simulink library "T_Sensor_Surface"  (Simulink 8.2)
settings: Solver=ode45  StartTime=0.0  StopTime=10.0  RelTol=1e-3
settings Model: Creator=lena.frank  LastModifiedBy=drhf

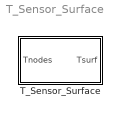
== system T_Sensor_Surface ==
  T_Sensor_Surface : Subsystem  mask(surface temperature sensor){pos=[0.1 0.4 0.5 0.9], tdel=1, t0=20}
      mask prompts: pos "relative position 0..1 (0 = bottom, 1 = top)"; tdel "delay-time in s"; t0 "initial temperature in degree centigrade"
      mask help:
      | Surface temperature sensor for a storage. The block breaks the algebraic loop when connecting the node temperature directly to the controller.
      | The relative position can be a vector for several sensors, for example [0.1 0.5 0.9]
      mask init:
      | tdel = max(tdel,0.01);
      | pos = max(0, min(pos, 1));
      mask Help: web(fullfile(path_carnot('help'),'T_Sensor_Surface.html'),'-helpbrowser')
      mask Display: plot(-10,0,110,100,[50,55,65,70,70,65,55,45,35,30,30,35,44,50,50],[50,50,60,70,80,90,100,100,90,80,70,60,50,50,-0],[60,40],[90,90],[50,50],[57,90])

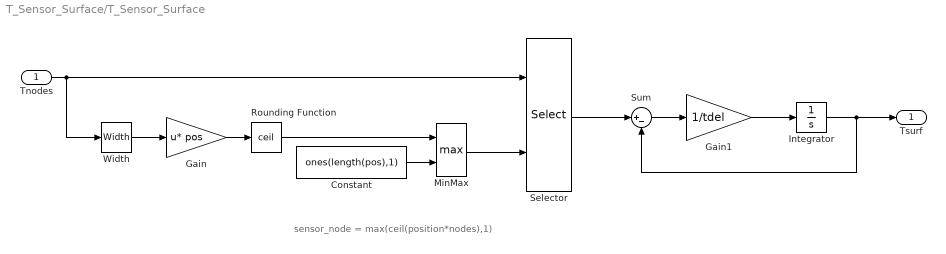
== system T_Sensor_Surface/T_Sensor_Surface ==
  note: sensor_node = max(ceil(position*nodes),1)
  Tnodes : Inport
  Constant : Constant  Value=ones(length(pos),1)
  Gain : Gain  Gain=pos  Multiplication=Matrix(u*K)
  Gain1 : Gain  Gain=1/tdel
  Integrator : Integrator  InitialCondition=t0
  MinMax : MinMax  Function=max  Inputs=2
  Rounding Function : Rounding  Operator=ceil
  Selector : Selector  IndexOptions=Index vector (port)  Indices=[1 3]  OutputSizes=1
  Sum : Sum  Inputs=|+-
  Width : Width
  Tsurf : Outport
  wires:
  Gain1/1 -> Integrator/1
  Width/1 -> Gain/1
  Tnodes/1 -> Width/1, Selector/1
  Sum/1 -> Gain1/1
  Integrator/1 -> Sum/2, Tsurf/1
  Selector/1 -> Sum/1
  Gain/1 -> Rounding Function/1
  Rounding Function/1 -> MinMax/1
  Constant/1 -> MinMax/2
  MinMax/1 -> Selector/2
